simulink model "DCmotor"  (R2022b)
settings: Solver=VariableStepAuto  StartTime=0.0  StopTime=10  RelTol=1e-3
values from neighbouring files (symbols this model uses):
  B = 0.00002    (= 2e-05)    [Parameters.m]
  J = 2.09e-5    (= 2.09e-05)    [Parameters.m]
  Kb = 0.042    [Parameters.m]
  Kt = 0.042    [Parameters.m]
  L = 1.16    [Parameters.m]
  R = 8.4    [Parameters.m]
  Tl = 0.0001    [Parameters.m]
settings Model: Creator=ParkJunHo  LastModifiedBy=ParkJunHo

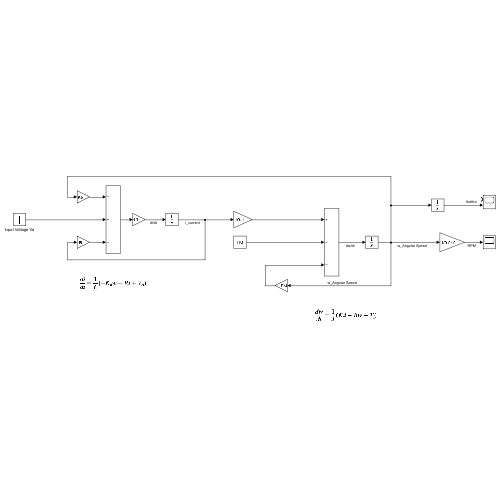
[thumbnail: Simulink's stored preview of the top-level diagram]
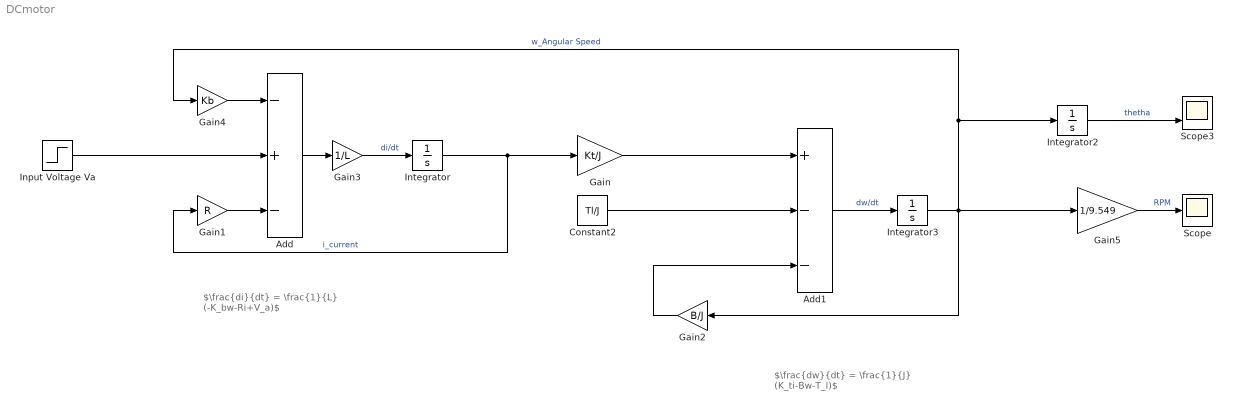
== system DCmotor ==
  note: $\frac{dw}{dt} = \frac{1}{J} (K_ti-Bw-T_l)$
  note: $\frac{di}{dt} = \frac{1}{L} (-K_bw-Ri+V_a)$
  Add : Sum  Inputs=-+-
  Add1 : Sum  Inputs=+--
  Constant2 : Constant  Value=Tl/J
  Gain : Gain  Gain=Kt/J
  Gain1 : Gain  Gain=R
  Gain2 : Gain  Gain=B/J
  Gain3 : Gain  Gain=1/L
  Gain4 : Gain  Gain=Kb
  Gain5 : Gain  Gain=1/9.549
  Input Voltage Va : Step  Time=5  Before=12  After=24  SampleTime=0
  Integrator : Integrator
  Integrator2 : Integrator
  Integrator3 : Integrator
  Scope : Scope
  Scope3 : Scope  NumInputPorts=2
  wires:
  Input Voltage Va/1 -> Add/2
  Gain3/1 -> Integrator/1  "di/dt"
  Constant2/1 -> Add1/2
  Gain4/1 -> Add/1
  Gain1/1 -> Add/3
  Integrator3/1 -> Gain4/1, Integrator2/1, Gain5/1, Gain2/1  "w_Angular Speed"
  Integrator/1 -> Gain/1, Gain1/1  "i_current"
  Add1/1 -> Integrator3/1  "dw/dt"
  Gain/1 -> Add1/1
  Integrator2/1 -> Scope3/2  "thetha"
  Add/1 -> Gain3/1
  Gain2/1 -> Add1/3
  Gain5/1 -> Scope/1  "RPM"
